simulink model "BT3"  (R2019a)
settings: Solver=ode5  StartTime=0.0  StopTime=12  FixedStep=0.001  RelTol=1e-3
libraries: fuzblock x1
settings Model: Creator=ASUS  LastModifiedBy=ASUS

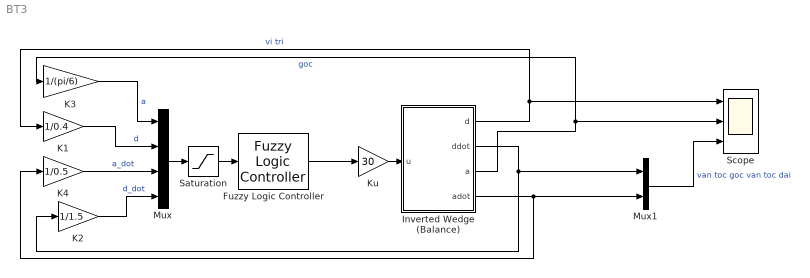
== system BT3 ==
  Fuzzy Logic Controller : fuzblock/Fuzzy Logic  Controller  FIS='bt3.fis'  OutputSampleNumber=101  DataType=double  FuzzifiedInputs=off  RuleFiringStrengths=off  RuleOutputs=off  AggregatedOutputs=off  SimulateUsing=Interpreted execution  OutOfRangeInputValueMessage=warning  NoRuleFiredMessage=warning  EmptyOutputFuzzySetMessage=warning
  "Inverted Wedge (Balance) " : Subsystem  mask{g=9.81, a=0.11, c=0.045, m_=0.49, M=3.3, J=0.42, km=5, b=5, d0=-0.35, ddot0=0.6, a0=0.5, adot0=-0.3}
  K1 : Gain  Gain=1/0.4
  K2 : Gain  Gain=1/1.5
  K3 : Gain  Gain=1/(pi/6)
  K4 : Gain  Gain=1/0.5
  Ku : Gain  Gain=30
  Mux : Mux
  Mux1 : Mux  Inputs=2
  Saturation : Saturate  UpperLimit=1  LowerLimit=-1
  Scope : Scope  NumInputPorts=3
  wires:
  "Inverted Wedge (Balance) "/1(d) -> K1/1, Scope/1  "vi tri"
  "Inverted Wedge (Balance) "/3(a) -> K3/1, Scope/2  "goc"
  "Inverted Wedge (Balance) "/4(adot) -> K4/1, Mux1/2
  Fuzzy Logic Controller/1 -> Ku/1
  "Inverted Wedge (Balance) "/2(ddot) -> K2/1, Mux1/1
  Mux/1 -> Saturation/1
  Saturation/1 -> Fuzzy Logic Controller/1
  Ku/1 -> "Inverted Wedge (Balance) "/1(u)
  Mux1/1 -> Scope/3  "van toc goc van toc dai"
  K3/1 -> Mux/1  "a"
  K1/1 -> Mux/2  "d"
  K2/1 -> Mux/4  "d_dot"
  K4/1 -> Mux/3  "a_dot"

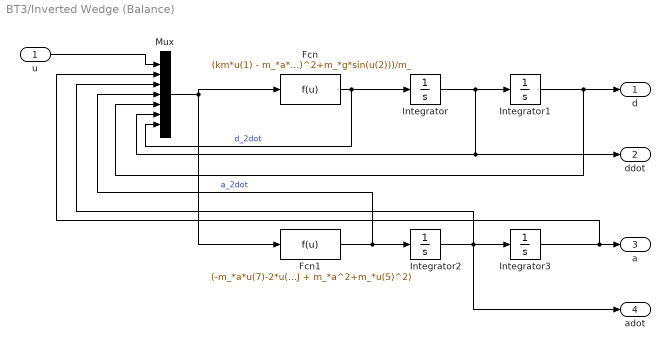
== system BT3/Inverted Wedge (Balance)  ==
  u : Inport
  Fcn : Fcn  Expr=(km*u(1) - m_*a*u(4)-b*u(6)+m_*u(5)*u(3)^2+m_*g*sin(u(2)))/m_
  Fcn1 : Fcn  Expr=(-m_*a*u(7)-2*u(3)*m_*u(5)*u(6)+m_*g*a*sin(u(2))+m_*g*u(5)*cos(u(2))+M*g*c*sin(u(2)))/(J + m_*a^2+m_*u(5)^2)
  Integrator : Integrator  InitialCondition=ddot0
  Integrator1 : Integrator  InitialCondition=d0
  Integrator2 : Integrator  InitialCondition=adot0
  Integrator3 : Integrator  InitialCondition=a0
  Mux : Mux  Inputs=7
  d : Outport
  ddot : Outport  Port=2
  a : Outport  Port=3
  adot : Outport  Port=4
  wires:
  u/1 -> Mux/1
  Fcn/1 -> Mux/7, Integrator/1  "d_2dot"
  Integrator/1 -> Mux/6, ddot/1, Integrator1/1
  Integrator1/1 -> Mux/5, d/1
  Mux/1 -> Fcn/1, Fcn1/1
  Integrator3/1 -> Mux/2, a/1
  Integrator2/1 -> Mux/3, Integrator3/1, adot/1
  Fcn1/1 -> Mux/4, Integrator2/1  "a_2dot"
